simulink model "Lab_08"  (R2023a)
settings: Solver=VariableStepAuto  StartTime=0.0  StopTime=10.0  RelTol=1e-3
libraries: dspquant2 x2
settings Model: Creator=fahim  LastModifiedBy=fahim

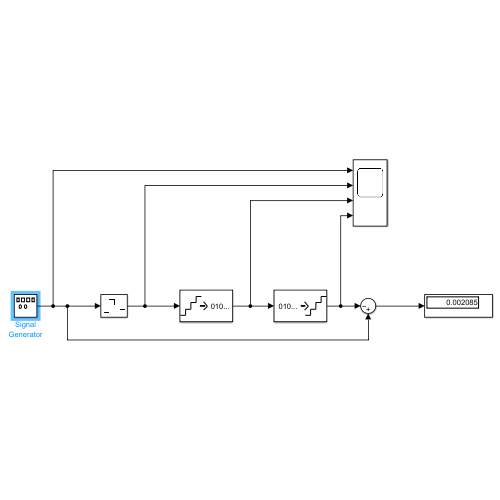
[thumbnail: Simulink's stored preview of the top-level diagram]
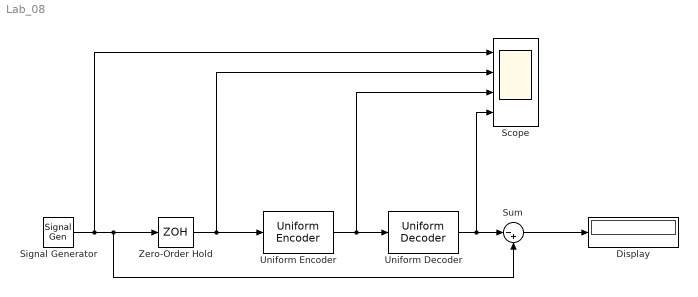
== system Lab_08 ==
  Display : Display
  Scope : Scope  NumInputPorts=4
  Signal Generator : SignalGenerator  WaveForm=sawtooth  Frequency=20  Units=rad/sec
  Sum : Sum  Inputs=|-+
  Uniform Decoder : dspquant2/Uniform Decoder  peak=1  bits=8  overflowMode=Saturate  otype=Double
  Uniform Encoder : dspquant2/Uniform Encoder  peak=1  bits=8  otype=Unsigned integer
  Zero-Order Hold : ZeroOrderHold  SampleTime=0.1
  wires:
  Signal Generator/1 -> Scope/1, Sum/2, Zero-Order Hold/1
  Zero-Order Hold/1 -> Scope/2, Uniform Encoder/1
  Uniform Encoder/1 -> Scope/3, Uniform Decoder/1
  Sum/1 -> Display/1
  Uniform Decoder/1 -> Scope/4, Sum/1
